simulink model "Cooling_System"  (R2019b)
settings: Solver=VariableStepAuto  StartTime=0.0  StopTime=3600  RelTol=1e-3
libraries: fl_lib x170, nesl_utility x49
(part 1 of 2)
settings Model: Creator=ZHOU Jinhan  LastModifiedBy=ZHOU Jinhan

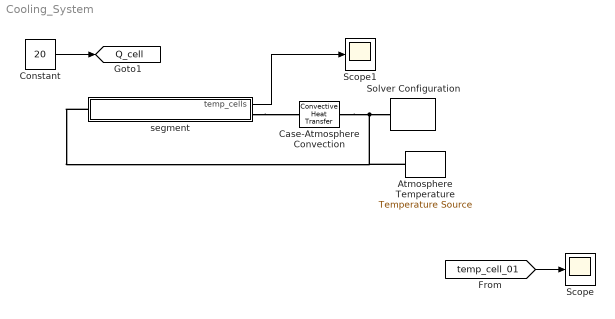
== system Cooling_System ==
  Atmosphere Temperature : fl_lib/Thermal/Thermal Sources/Temperature Source  temperature=25 degC
      settings: SourceProductName=Simscape
  Case-Atmosphere Convection : fl_lib/Thermal/Thermal Elements/Convective Heat Transfer  area=2160 cm^2  heat_tr_coeff=50 W/(m^2 * K)  T_specify=off  T_priority=None  T=0 K  T_nominal_specify=off  T_nominal_unit=K  T_nominal_value=1  Q_specify=off  Q_priority=None  Q=0 W  Q_nominal_specify=off  Q_nominal_unit=W  Q_nominal_value=1
  Constant : Constant  Value=20
  Scope : Scope
  Scope1 : Scope
  Solver Configuration : nesl_utility/Solver Configuration  PhysicalDomain=network_engine_domain  SubClassName=solver  LeftPortType=input  RightPortType=generic  Tones=[]  Harmonics=[]  SimulateNoise=off  Profile=off  UseLocalSampling=off  EnableSwitchedLinearOptims=on  FrequencyDomain=off  UseCCode=off  RelTol=0.001  AbsTol=1e-06  MinStep=1e-09  ToWorkspace=off  RevertToSquareIcSolve=off  NumHomotopyIterations=100  PhasorMode=off  PhasorModeNumHarmonics=1  DoDC=off  ResidualTolerance=1e-9  UseLocalSolver=off  LocalSolverChoice=NE_BACKWARD_EULER_ADVANCER  LocalSolverSampleTime=.001  DoFixedCost=off  MaxNonlinIter=3  MaxModeIter=2  LinearAlgebra=auto  EquationFormulation=NE_TIME_EF  DelaysMemoryBudget=1024  AutomaticFiltering=on  FilteringTimeConstant=0.001  PartitionStorageMethod=AS_NEEDED  PartitionMemoryBudget=1024  PartitionMethod=FAST
  segment : Subsystem
  tag scope: Q_cell=global
  wires:
  Constant/1 -> [Q_cell]
  [temp_cell_01] -> Scope/1
  segment/1(temp_cells) -> Scope1/1
  connections:
  segment/RConn1 -- Case-Atmosphere Convection/LConn1
  Case-Atmosphere Convection/RConn1 -- segment/LConn1 -- Atmosphere Temperature/LConn1 -- Solver Configuration/RConn1

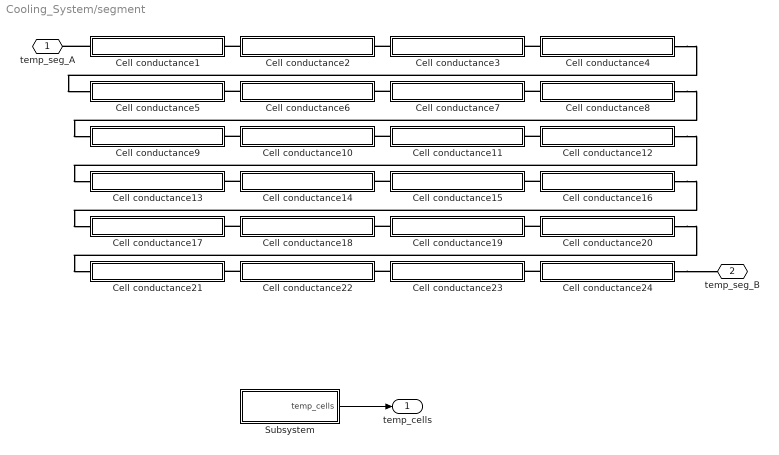
== system Cooling_System/segment ==
  Cell conductance1 : Subsystem
  Cell conductance10 : Subsystem
  Cell conductance11 : Subsystem
  Cell conductance12 : Subsystem
  Cell conductance13 : Subsystem
  Cell conductance14 : Subsystem
  Cell conductance15 : Subsystem
  Cell conductance16 : Subsystem
  Cell conductance17 : Subsystem
  Cell conductance18 : Subsystem
  "Cell conductance19 " : Subsystem
  Cell conductance2 : Subsystem
  Cell conductance20 : Subsystem
  Cell conductance21 : Subsystem
  Cell conductance22 : Subsystem
  Cell conductance23 : Subsystem
  Cell conductance24 : Subsystem
  Cell conductance3 : Subsystem
  Cell conductance4 : Subsystem
  Cell conductance5 : Subsystem
  Cell conductance6 : Subsystem
  Cell conductance7 : Subsystem
  Cell conductance8 : Subsystem
  Cell conductance9 : Subsystem
  Subsystem : Subsystem
  temp_seg_A : PMIOPort  Side=Left
  temp_seg_B : PMIOPort  Port=2  Side=Right
  temp_cells : Outport
  wires:
  Subsystem/1(temp_cells) -> temp_cells/1
  connections:
  Cell conductance2/LConn1 -- Cell conductance1/RConn1
  Cell conductance1/LConn1 -- temp_seg_A/RConn1
  Cell conductance24/RConn1 -- temp_seg_B/RConn1
  Cell conductance3/LConn1 -- Cell conductance2/RConn1
  Cell conductance4/LConn1 -- Cell conductance3/RConn1
  Cell conductance6/LConn1 -- Cell conductance5/RConn1
  Cell conductance7/LConn1 -- Cell conductance6/RConn1
  Cell conductance8/LConn1 -- Cell conductance7/RConn1
  Cell conductance10/LConn1 -- Cell conductance9/RConn1
  Cell conductance11/LConn1 -- Cell conductance10/RConn1
  Cell conductance12/LConn1 -- Cell conductance11/RConn1
  Cell conductance24/LConn1 -- Cell conductance23/RConn1
  Cell conductance23/LConn1 -- Cell conductance22/RConn1
  Cell conductance14/LConn1 -- Cell conductance13/RConn1
  Cell conductance18/LConn1 -- Cell conductance17/RConn1
  Cell conductance15/LConn1 -- Cell conductance14/RConn1
  Cell conductance16/LConn1 -- Cell conductance15/RConn1
  "Cell conductance19 "/LConn1 -- Cell conductance18/RConn1
  Cell conductance22/LConn1 -- Cell conductance21/RConn1
  Cell conductance20/LConn1 -- "Cell conductance19 "/RConn1
  Cell conductance4/RConn1 -- Cell conductance5/LConn1
  Cell conductance8/RConn1 -- Cell conductance9/LConn1
  Cell conductance12/RConn1 -- Cell conductance13/LConn1
  Cell conductance16/RConn1 -- Cell conductance17/LConn1
  Cell conductance20/RConn1 -- Cell conductance21/LConn1

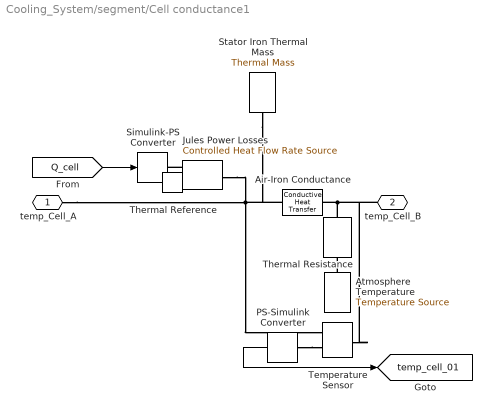
== system Cooling_System/segment/Cell conductance1 ==
  Air-Iron Conductance : fl_lib/Thermal/Thermal Elements/Conductive Heat Transfer  area=0.014 m^2  thickness=2 mm  th_cond=0.0257 W/(m*K)  T_specify=off  T_priority=None  T=0 K  T_nominal_specify=off  T_nominal_unit=K  T_nominal_value=1  Q_specify=off  Q_priority=None  Q=0 W  Q_nominal_specify=off  Q_nominal_unit=W  Q_nominal_value=1
      settings: SourceProductName=Simscape
  Atmosphere Temperature : fl_lib/Thermal/Thermal Sources/Temperature Source  temperature=300 K
      settings: SourceProductName=Simscape
  Jules Power Losses : fl_lib/Thermal/Thermal Sources/Controlled Heat Flow Rate Source
      settings: SourceProductName=Simscape
  PS-Simulink Converter : nesl_utility/PS-Simulink Converter  PhysicalDomain=network_engine_domain  SubClassName=ps_output  LeftPortType=input  RightPortType=output  PseudoPeriodic=off  Frequencies=[]  Unit=1  AffineConversion=off
  Simulink-PS Converter : nesl_utility/Simulink-PS Converter  PhysicalDomain=network_engine_domain  SubClassName=ps_input  LeftPortType=input  RightPortType=output  PseudoPeriodic=off  Frequencies=[]  NoiseDistribution=none  NoiseParameters=[]  Unit=W  AffineConversion=off  FilteringAndDerivatives=zero  SimscapeFilterOrder=1  InputFilterTimeConstant=.001  UdotUserProvided=[]
  Stator Iron Thermal Mass : fl_lib/Thermal/Thermal Elements/Thermal Mass  mass=0.3 kg  sp_heat=460 J/kg/K  T_specify=off  T_priority=High  T=300 K  T_nominal_specify=off  T_nominal_unit=K  T_nominal_value=1  Q_specify=off  Q_priority=None  Q=0 W  Q_nominal_specify=off  Q_nominal_unit=W  Q_nominal_value=1
  Temperature Sensor : fl_lib/Thermal/Thermal Sensors/Temperature Sensor
  Thermal Reference : fl_lib/Thermal/Thermal Elements/Thermal Reference
  Thermal Resistance : fl_lib/Thermal/Thermal Elements/Thermal Resistance  resistance=1/(1.006*1.202*0.028*50.4/60*1000) K/W  T_specify=off  T_priority=None  T=0 K  T_nominal_specify=off  T_nominal_unit=K  T_nominal_value=1  Q_specify=off  Q_priority=None  Q=0 W  Q_nominal_specify=off  Q_nominal_unit=W  Q_nominal_value=1
      settings: SourceProductName=Simscape  SourceProductBaseCode=SS
  temp_Cell_A : PMIOPort  Side=Left
  temp_Cell_B : PMIOPort  Port=2  Side=Right
  tag scope: temp_cell_01=global
  wires:
  [Q_cell] -> Simulink-PS Converter/1
  PS-Simulink Converter/1 -> [temp_cell_01]
  connections:
  temp_Cell_A/RConn1 -- Stator Iron Thermal Mass/LConn1 -- Air-Iron Conductance/LConn1 -- Jules Power Losses/LConn1 -- Temperature Sensor/RConn1
  Air-Iron Conductance/RConn1 -- Temperature Sensor/LConn1 -- temp_Cell_B/RConn1 -- Thermal Resistance/LConn1
  Atmosphere Temperature/LConn1 -- Thermal Resistance/RConn1
  Jules Power Losses/RConn1 -- Simulink-PS Converter/RConn1
  PS-Simulink Converter/LConn1 -- Temperature Sensor/RConn2
  Thermal Reference/LConn1 -- Jules Power Losses/RConn2

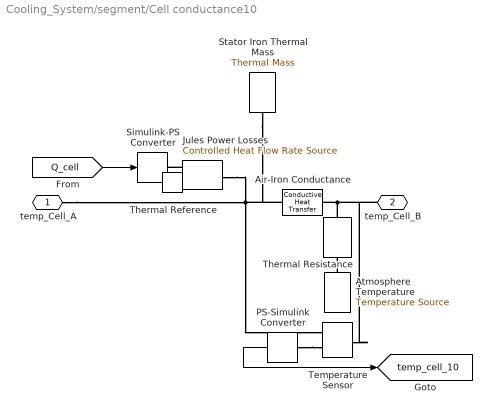
== system Cooling_System/segment/Cell conductance10 ==
  Air-Iron Conductance : fl_lib/Thermal/Thermal Elements/Conductive Heat Transfer  area=0.014 m^2  thickness=2 mm  th_cond=0.0257 W/(m*K)  T_specify=off  T_priority=None  T=0 K  T_nominal_specify=off  T_nominal_unit=K  T_nominal_value=1  Q_specify=off  Q_priority=None  Q=0 W  Q_nominal_specify=off  Q_nominal_unit=W  Q_nominal_value=1
      settings: SourceProductName=Simscape
  Atmosphere Temperature : fl_lib/Thermal/Thermal Sources/Temperature Source  temperature=300 K
      settings: SourceProductName=Simscape
  Jules Power Losses : fl_lib/Thermal/Thermal Sources/Controlled Heat Flow Rate Source
      settings: SourceProductName=Simscape
  PS-Simulink Converter : nesl_utility/PS-Simulink Converter  PhysicalDomain=network_engine_domain  SubClassName=ps_output  LeftPortType=input  RightPortType=output  PseudoPeriodic=off  Frequencies=[]  Unit=1  AffineConversion=off
  Simulink-PS Converter : nesl_utility/Simulink-PS Converter  PhysicalDomain=network_engine_domain  SubClassName=ps_input  LeftPortType=input  RightPortType=output  PseudoPeriodic=off  Frequencies=[]  NoiseDistribution=none  NoiseParameters=[]  Unit=W  AffineConversion=off  FilteringAndDerivatives=zero  SimscapeFilterOrder=1  InputFilterTimeConstant=.001  UdotUserProvided=[]
  Stator Iron Thermal Mass : fl_lib/Thermal/Thermal Elements/Thermal Mass  mass=0.3 kg  sp_heat=460 J/kg/K  T_specify=off  T_priority=High  T=300 K  T_nominal_specify=off  T_nominal_unit=K  T_nominal_value=1  Q_specify=off  Q_priority=None  Q=0 W  Q_nominal_specify=off  Q_nominal_unit=W  Q_nominal_value=1
  Temperature Sensor : fl_lib/Thermal/Thermal Sensors/Temperature Sensor
  Thermal Reference : fl_lib/Thermal/Thermal Elements/Thermal Reference
  Thermal Resistance : fl_lib/Thermal/Thermal Elements/Thermal Resistance  resistance=1/(1.006*1.202*0.028*50.4/60*1000) K/W  T_specify=off  T_priority=None  T=0 K  T_nominal_specify=off  T_nominal_unit=K  T_nominal_value=1  Q_specify=off  Q_priority=None  Q=0 W  Q_nominal_specify=off  Q_nominal_unit=W  Q_nominal_value=1
      settings: SourceProductName=Simscape  SourceProductBaseCode=SS
  temp_Cell_A : PMIOPort  Side=Left
  temp_Cell_B : PMIOPort  Port=2  Side=Right
  tag scope: temp_cell_10=global
  wires:
  [Q_cell] -> Simulink-PS Converter/1
  PS-Simulink Converter/1 -> [temp_cell_10]
  connections:
  Jules Power Losses/LConn1 -- temp_Cell_A/RConn1 -- Temperature Sensor/RConn1 -- Stator Iron Thermal Mass/LConn1 -- Air-Iron Conductance/LConn1
  Air-Iron Conductance/RConn1 -- Thermal Resistance/LConn1 -- temp_Cell_B/RConn1 -- Temperature Sensor/LConn1
  Atmosphere Temperature/LConn1 -- Thermal Resistance/RConn1
  Jules Power Losses/RConn1 -- Simulink-PS Converter/RConn1
  PS-Simulink Converter/LConn1 -- Temperature Sensor/RConn2
  Thermal Reference/LConn1 -- Jules Power Losses/RConn2

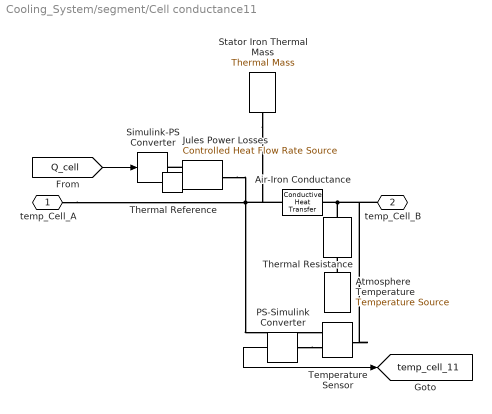
== system Cooling_System/segment/Cell conductance11 ==
  Air-Iron Conductance : fl_lib/Thermal/Thermal Elements/Conductive Heat Transfer  area=0.014 m^2  thickness=2 mm  th_cond=0.0257 W/(m*K)  T_specify=off  T_priority=None  T=0 K  T_nominal_specify=off  T_nominal_unit=K  T_nominal_value=1  Q_specify=off  Q_priority=None  Q=0 W  Q_nominal_specify=off  Q_nominal_unit=W  Q_nominal_value=1
      settings: SourceProductName=Simscape
  Atmosphere Temperature : fl_lib/Thermal/Thermal Sources/Temperature Source  temperature=300 K
      settings: SourceProductName=Simscape
  Jules Power Losses : fl_lib/Thermal/Thermal Sources/Controlled Heat Flow Rate Source
      settings: SourceProductName=Simscape
  PS-Simulink Converter : nesl_utility/PS-Simulink Converter  PhysicalDomain=network_engine_domain  SubClassName=ps_output  LeftPortType=input  RightPortType=output  PseudoPeriodic=off  Frequencies=[]  Unit=1  AffineConversion=off
  Simulink-PS Converter : nesl_utility/Simulink-PS Converter  PhysicalDomain=network_engine_domain  SubClassName=ps_input  LeftPortType=input  RightPortType=output  PseudoPeriodic=off  Frequencies=[]  NoiseDistribution=none  NoiseParameters=[]  Unit=W  AffineConversion=off  FilteringAndDerivatives=zero  SimscapeFilterOrder=1  InputFilterTimeConstant=.001  UdotUserProvided=[]
  Stator Iron Thermal Mass : fl_lib/Thermal/Thermal Elements/Thermal Mass  mass=0.3 kg  sp_heat=460 J/kg/K  T_specify=off  T_priority=High  T=300 K  T_nominal_specify=off  T_nominal_unit=K  T_nominal_value=1  Q_specify=off  Q_priority=None  Q=0 W  Q_nominal_specify=off  Q_nominal_unit=W  Q_nominal_value=1
  Temperature Sensor : fl_lib/Thermal/Thermal Sensors/Temperature Sensor
  Thermal Reference : fl_lib/Thermal/Thermal Elements/Thermal Reference
  Thermal Resistance : fl_lib/Thermal/Thermal Elements/Thermal Resistance  resistance=1/(1.006*1.202*0.028*50.4/60*1000) K/W  T_specify=off  T_priority=None  T=0 K  T_nominal_specify=off  T_nominal_unit=K  T_nominal_value=1  Q_specify=off  Q_priority=None  Q=0 W  Q_nominal_specify=off  Q_nominal_unit=W  Q_nominal_value=1
      settings: SourceProductName=Simscape  SourceProductBaseCode=SS
  temp_Cell_A : PMIOPort  Side=Left
  temp_Cell_B : PMIOPort  Port=2  Side=Right
  tag scope: temp_cell_11=global
  wires:
  [Q_cell] -> Simulink-PS Converter/1
  PS-Simulink Converter/1 -> [temp_cell_11]
  connections:
  Jules Power Losses/LConn1 -- temp_Cell_A/RConn1 -- Temperature Sensor/RConn1 -- Stator Iron Thermal Mass/LConn1 -- Air-Iron Conductance/LConn1
  Air-Iron Conductance/RConn1 -- Thermal Resistance/LConn1 -- temp_Cell_B/RConn1 -- Temperature Sensor/LConn1
  Atmosphere Temperature/LConn1 -- Thermal Resistance/RConn1
  Jules Power Losses/RConn1 -- Simulink-PS Converter/RConn1
  PS-Simulink Converter/LConn1 -- Temperature Sensor/RConn2
  Thermal Reference/LConn1 -- Jules Power Losses/RConn2

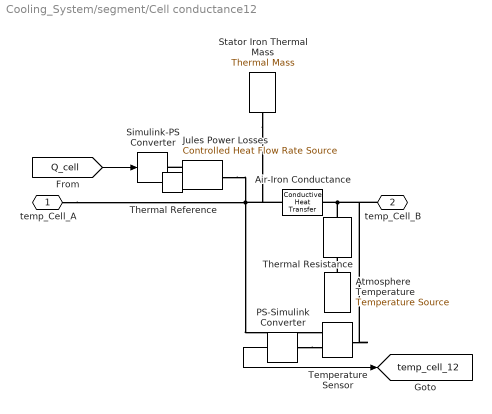
== system Cooling_System/segment/Cell conductance12 ==
  Air-Iron Conductance : fl_lib/Thermal/Thermal Elements/Conductive Heat Transfer  area=0.014 m^2  thickness=2 mm  th_cond=0.0257 W/(m*K)  T_specify=off  T_priority=None  T=0 K  T_nominal_specify=off  T_nominal_unit=K  T_nominal_value=1  Q_specify=off  Q_priority=None  Q=0 W  Q_nominal_specify=off  Q_nominal_unit=W  Q_nominal_value=1
      settings: SourceProductName=Simscape
  Atmosphere Temperature : fl_lib/Thermal/Thermal Sources/Temperature Source  temperature=300 K
      settings: SourceProductName=Simscape
  Jules Power Losses : fl_lib/Thermal/Thermal Sources/Controlled Heat Flow Rate Source
      settings: SourceProductName=Simscape
  PS-Simulink Converter : nesl_utility/PS-Simulink Converter  PhysicalDomain=network_engine_domain  SubClassName=ps_output  LeftPortType=input  RightPortType=output  PseudoPeriodic=off  Frequencies=[]  Unit=1  AffineConversion=off
  Simulink-PS Converter : nesl_utility/Simulink-PS Converter  PhysicalDomain=network_engine_domain  SubClassName=ps_input  LeftPortType=input  RightPortType=output  PseudoPeriodic=off  Frequencies=[]  NoiseDistribution=none  NoiseParameters=[]  Unit=W  AffineConversion=off  FilteringAndDerivatives=zero  SimscapeFilterOrder=1  InputFilterTimeConstant=.001  UdotUserProvided=[]
  Stator Iron Thermal Mass : fl_lib/Thermal/Thermal Elements/Thermal Mass  mass=0.3 kg  sp_heat=460 J/kg/K  T_specify=off  T_priority=High  T=300 K  T_nominal_specify=off  T_nominal_unit=K  T_nominal_value=1  Q_specify=off  Q_priority=None  Q=0 W  Q_nominal_specify=off  Q_nominal_unit=W  Q_nominal_value=1
  Temperature Sensor : fl_lib/Thermal/Thermal Sensors/Temperature Sensor
  Thermal Reference : fl_lib/Thermal/Thermal Elements/Thermal Reference
  Thermal Resistance : fl_lib/Thermal/Thermal Elements/Thermal Resistance  resistance=1/(1.006*1.202*0.028*50.4/60*1000) K/W  T_specify=off  T_priority=None  T=0 K  T_nominal_specify=off  T_nominal_unit=K  T_nominal_value=1  Q_specify=off  Q_priority=None  Q=0 W  Q_nominal_specify=off  Q_nominal_unit=W  Q_nominal_value=1
      settings: SourceProductName=Simscape  SourceProductBaseCode=SS
  temp_Cell_A : PMIOPort  Side=Left
  temp_Cell_B : PMIOPort  Port=2  Side=Right
  tag scope: temp_cell_12=global
  wires:
  [Q_cell] -> Simulink-PS Converter/1
  PS-Simulink Converter/1 -> [temp_cell_12]
  connections:
  Jules Power Losses/LConn1 -- temp_Cell_A/RConn1 -- Temperature Sensor/RConn1 -- Stator Iron Thermal Mass/LConn1 -- Air-Iron Conductance/LConn1
  Air-Iron Conductance/RConn1 -- Thermal Resistance/LConn1 -- temp_Cell_B/RConn1 -- Temperature Sensor/LConn1
  Atmosphere Temperature/LConn1 -- Thermal Resistance/RConn1
  Jules Power Losses/RConn1 -- Simulink-PS Converter/RConn1
  PS-Simulink Converter/LConn1 -- Temperature Sensor/RConn2
  Thermal Reference/LConn1 -- Jules Power Losses/RConn2

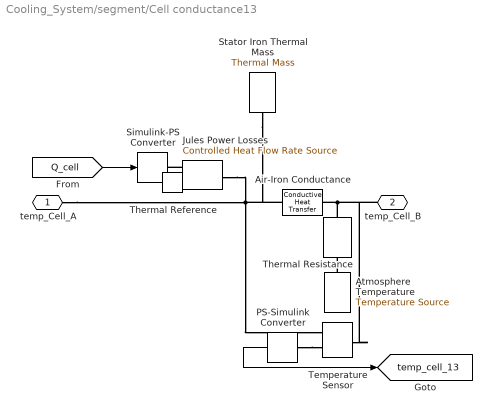
== system Cooling_System/segment/Cell conductance13 ==
  Air-Iron Conductance : fl_lib/Thermal/Thermal Elements/Conductive Heat Transfer  area=0.014 m^2  thickness=2 mm  th_cond=0.0257 W/(m*K)  T_specify=off  T_priority=None  T=0 K  T_nominal_specify=off  T_nominal_unit=K  T_nominal_value=1  Q_specify=off  Q_priority=None  Q=0 W  Q_nominal_specify=off  Q_nominal_unit=W  Q_nominal_value=1
      settings: SourceProductName=Simscape
  Atmosphere Temperature : fl_lib/Thermal/Thermal Sources/Temperature Source  temperature=300 K
      settings: SourceProductName=Simscape
  Jules Power Losses : fl_lib/Thermal/Thermal Sources/Controlled Heat Flow Rate Source
      settings: SourceProductName=Simscape
  PS-Simulink Converter : nesl_utility/PS-Simulink Converter  PhysicalDomain=network_engine_domain  SubClassName=ps_output  LeftPortType=input  RightPortType=output  PseudoPeriodic=off  Frequencies=[]  Unit=1  AffineConversion=off
  Simulink-PS Converter : nesl_utility/Simulink-PS Converter  PhysicalDomain=network_engine_domain  SubClassName=ps_input  LeftPortType=input  RightPortType=output  PseudoPeriodic=off  Frequencies=[]  NoiseDistribution=none  NoiseParameters=[]  Unit=W  AffineConversion=off  FilteringAndDerivatives=zero  SimscapeFilterOrder=1  InputFilterTimeConstant=.001  UdotUserProvided=[]
  Stator Iron Thermal Mass : fl_lib/Thermal/Thermal Elements/Thermal Mass  mass=0.3 kg  sp_heat=460 J/kg/K  T_specify=off  T_priority=High  T=300 K  T_nominal_specify=off  T_nominal_unit=K  T_nominal_value=1  Q_specify=off  Q_priority=None  Q=0 W  Q_nominal_specify=off  Q_nominal_unit=W  Q_nominal_value=1
  Temperature Sensor : fl_lib/Thermal/Thermal Sensors/Temperature Sensor
  Thermal Reference : fl_lib/Thermal/Thermal Elements/Thermal Reference
  Thermal Resistance : fl_lib/Thermal/Thermal Elements/Thermal Resistance  resistance=1/(1.006*1.202*0.028*50.4/60*1000) K/W  T_specify=off  T_priority=None  T=0 K  T_nominal_specify=off  T_nominal_unit=K  T_nominal_value=1  Q_specify=off  Q_priority=None  Q=0 W  Q_nominal_specify=off  Q_nominal_unit=W  Q_nominal_value=1
      settings: SourceProductName=Simscape  SourceProductBaseCode=SS
  temp_Cell_A : PMIOPort  Side=Left
  temp_Cell_B : PMIOPort  Port=2  Side=Right
  tag scope: temp_cell_13=global
  wires:
  [Q_cell] -> Simulink-PS Converter/1
  PS-Simulink Converter/1 -> [temp_cell_13]
  connections:
  Jules Power Losses/LConn1 -- temp_Cell_A/RConn1 -- Temperature Sensor/RConn1 -- Stator Iron Thermal Mass/LConn1 -- Air-Iron Conductance/LConn1
  Air-Iron Conductance/RConn1 -- Thermal Resistance/LConn1 -- temp_Cell_B/RConn1 -- Temperature Sensor/LConn1
  Atmosphere Temperature/LConn1 -- Thermal Resistance/RConn1
  Jules Power Losses/RConn1 -- Simulink-PS Converter/RConn1
  PS-Simulink Converter/LConn1 -- Temperature Sensor/RConn2
  Thermal Reference/LConn1 -- Jules Power Losses/RConn2

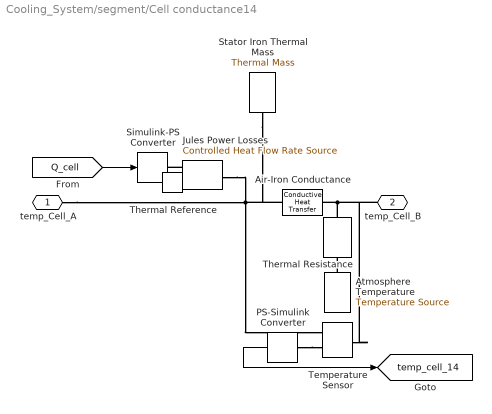
== system Cooling_System/segment/Cell conductance14 ==
  Air-Iron Conductance : fl_lib/Thermal/Thermal Elements/Conductive Heat Transfer  area=0.014 m^2  thickness=2 mm  th_cond=0.0257 W/(m*K)  T_specify=off  T_priority=None  T=0 K  T_nominal_specify=off  T_nominal_unit=K  T_nominal_value=1  Q_specify=off  Q_priority=None  Q=0 W  Q_nominal_specify=off  Q_nominal_unit=W  Q_nominal_value=1
      settings: SourceProductName=Simscape
  Atmosphere Temperature : fl_lib/Thermal/Thermal Sources/Temperature Source  temperature=300 K
      settings: SourceProductName=Simscape
  Jules Power Losses : fl_lib/Thermal/Thermal Sources/Controlled Heat Flow Rate Source
      settings: SourceProductName=Simscape
  PS-Simulink Converter : nesl_utility/PS-Simulink Converter  PhysicalDomain=network_engine_domain  SubClassName=ps_output  LeftPortType=input  RightPortType=output  PseudoPeriodic=off  Frequencies=[]  Unit=1  AffineConversion=off
  Simulink-PS Converter : nesl_utility/Simulink-PS Converter  PhysicalDomain=network_engine_domain  SubClassName=ps_input  LeftPortType=input  RightPortType=output  PseudoPeriodic=off  Frequencies=[]  NoiseDistribution=none  NoiseParameters=[]  Unit=W  AffineConversion=off  FilteringAndDerivatives=zero  SimscapeFilterOrder=1  InputFilterTimeConstant=.001  UdotUserProvided=[]
  Stator Iron Thermal Mass : fl_lib/Thermal/Thermal Elements/Thermal Mass  mass=0.3 kg  sp_heat=460 J/kg/K  T_specify=off  T_priority=High  T=300 K  T_nominal_specify=off  T_nominal_unit=K  T_nominal_value=1  Q_specify=off  Q_priority=None  Q=0 W  Q_nominal_specify=off  Q_nominal_unit=W  Q_nominal_value=1
  Temperature Sensor : fl_lib/Thermal/Thermal Sensors/Temperature Sensor
  Thermal Reference : fl_lib/Thermal/Thermal Elements/Thermal Reference
  Thermal Resistance : fl_lib/Thermal/Thermal Elements/Thermal Resistance  resistance=1/(1.006*1.202*0.028*50.4/60*1000) K/W  T_specify=off  T_priority=None  T=0 K  T_nominal_specify=off  T_nominal_unit=K  T_nominal_value=1  Q_specify=off  Q_priority=None  Q=0 W  Q_nominal_specify=off  Q_nominal_unit=W  Q_nominal_value=1
      settings: SourceProductName=Simscape  SourceProductBaseCode=SS
  temp_Cell_A : PMIOPort  Side=Left
  temp_Cell_B : PMIOPort  Port=2  Side=Right
  tag scope: temp_cell_14=global
  wires:
  [Q_cell] -> Simulink-PS Converter/1
  PS-Simulink Converter/1 -> [temp_cell_14]
  connections:
  Jules Power Losses/LConn1 -- temp_Cell_A/RConn1 -- Temperature Sensor/RConn1 -- Stator Iron Thermal Mass/LConn1 -- Air-Iron Conductance/LConn1
  Air-Iron Conductance/RConn1 -- Thermal Resistance/LConn1 -- temp_Cell_B/RConn1 -- Temperature Sensor/LConn1
  Atmosphere Temperature/LConn1 -- Thermal Resistance/RConn1
  Jules Power Losses/RConn1 -- Simulink-PS Converter/RConn1
  PS-Simulink Converter/LConn1 -- Temperature Sensor/RConn2
  Thermal Reference/LConn1 -- Jules Power Losses/RConn2

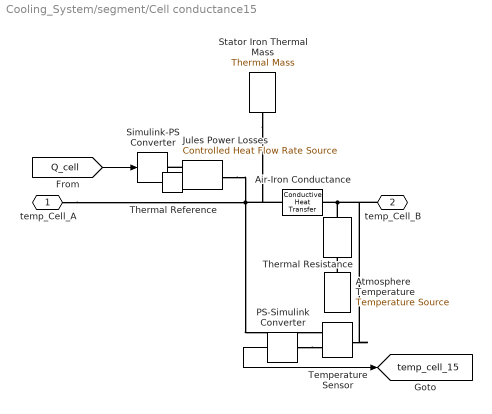
== system Cooling_System/segment/Cell conductance15 ==
  Air-Iron Conductance : fl_lib/Thermal/Thermal Elements/Conductive Heat Transfer  area=0.014 m^2  thickness=2 mm  th_cond=0.0257 W/(m*K)  T_specify=off  T_priority=None  T=0 K  T_nominal_specify=off  T_nominal_unit=K  T_nominal_value=1  Q_specify=off  Q_priority=None  Q=0 W  Q_nominal_specify=off  Q_nominal_unit=W  Q_nominal_value=1
      settings: SourceProductName=Simscape
  Atmosphere Temperature : fl_lib/Thermal/Thermal Sources/Temperature Source  temperature=300 K
      settings: SourceProductName=Simscape
  Jules Power Losses : fl_lib/Thermal/Thermal Sources/Controlled Heat Flow Rate Source
      settings: SourceProductName=Simscape
  PS-Simulink Converter : nesl_utility/PS-Simulink Converter  PhysicalDomain=network_engine_domain  SubClassName=ps_output  LeftPortType=input  RightPortType=output  PseudoPeriodic=off  Frequencies=[]  Unit=1  AffineConversion=off
  Simulink-PS Converter : nesl_utility/Simulink-PS Converter  PhysicalDomain=network_engine_domain  SubClassName=ps_input  LeftPortType=input  RightPortType=output  PseudoPeriodic=off  Frequencies=[]  NoiseDistribution=none  NoiseParameters=[]  Unit=W  AffineConversion=off  FilteringAndDerivatives=zero  SimscapeFilterOrder=1  InputFilterTimeConstant=.001  UdotUserProvided=[]
  Stator Iron Thermal Mass : fl_lib/Thermal/Thermal Elements/Thermal Mass  mass=0.3 kg  sp_heat=460 J/kg/K  T_specify=off  T_priority=High  T=300 K  T_nominal_specify=off  T_nominal_unit=K  T_nominal_value=1  Q_specify=off  Q_priority=None  Q=0 W  Q_nominal_specify=off  Q_nominal_unit=W  Q_nominal_value=1
  Temperature Sensor : fl_lib/Thermal/Thermal Sensors/Temperature Sensor
  Thermal Reference : fl_lib/Thermal/Thermal Elements/Thermal Reference
  Thermal Resistance : fl_lib/Thermal/Thermal Elements/Thermal Resistance  resistance=1/(1.006*1.202*0.028*50.4/60*1000) K/W  T_specify=off  T_priority=None  T=0 K  T_nominal_specify=off  T_nominal_unit=K  T_nominal_value=1  Q_specify=off  Q_priority=None  Q=0 W  Q_nominal_specify=off  Q_nominal_unit=W  Q_nominal_value=1
      settings: SourceProductName=Simscape  SourceProductBaseCode=SS
  temp_Cell_A : PMIOPort  Side=Left
  temp_Cell_B : PMIOPort  Port=2  Side=Right
  tag scope: temp_cell_15=global
  wires:
  [Q_cell] -> Simulink-PS Converter/1
  PS-Simulink Converter/1 -> [temp_cell_15]
  connections:
  Jules Power Losses/LConn1 -- temp_Cell_A/RConn1 -- Temperature Sensor/RConn1 -- Stator Iron Thermal Mass/LConn1 -- Air-Iron Conductance/LConn1
  Air-Iron Conductance/RConn1 -- Thermal Resistance/LConn1 -- temp_Cell_B/RConn1 -- Temperature Sensor/LConn1
  Atmosphere Temperature/LConn1 -- Thermal Resistance/RConn1
  Jules Power Losses/RConn1 -- Simulink-PS Converter/RConn1
  PS-Simulink Converter/LConn1 -- Temperature Sensor/RConn2
  Thermal Reference/LConn1 -- Jules Power Losses/RConn2

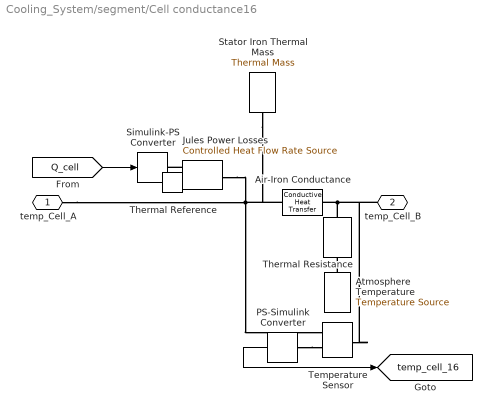
== system Cooling_System/segment/Cell conductance16 ==
  Air-Iron Conductance : fl_lib/Thermal/Thermal Elements/Conductive Heat Transfer  area=0.014 m^2  thickness=2 mm  th_cond=0.0257 W/(m*K)  T_specify=off  T_priority=None  T=0 K  T_nominal_specify=off  T_nominal_unit=K  T_nominal_value=1  Q_specify=off  Q_priority=None  Q=0 W  Q_nominal_specify=off  Q_nominal_unit=W  Q_nominal_value=1
      settings: SourceProductName=Simscape
  Atmosphere Temperature : fl_lib/Thermal/Thermal Sources/Temperature Source  temperature=300 K
      settings: SourceProductName=Simscape
  Jules Power Losses : fl_lib/Thermal/Thermal Sources/Controlled Heat Flow Rate Source
      settings: SourceProductName=Simscape
  PS-Simulink Converter : nesl_utility/PS-Simulink Converter  PhysicalDomain=network_engine_domain  SubClassName=ps_output  LeftPortType=input  RightPortType=output  PseudoPeriodic=off  Frequencies=[]  Unit=1  AffineConversion=off
  Simulink-PS Converter : nesl_utility/Simulink-PS Converter  PhysicalDomain=network_engine_domain  SubClassName=ps_input  LeftPortType=input  RightPortType=output  PseudoPeriodic=off  Frequencies=[]  NoiseDistribution=none  NoiseParameters=[]  Unit=W  AffineConversion=off  FilteringAndDerivatives=zero  SimscapeFilterOrder=1  InputFilterTimeConstant=.001  UdotUserProvided=[]
  Stator Iron Thermal Mass : fl_lib/Thermal/Thermal Elements/Thermal Mass  mass=0.3 kg  sp_heat=460 J/kg/K  T_specify=off  T_priority=High  T=300 K  T_nominal_specify=off  T_nominal_unit=K  T_nominal_value=1  Q_specify=off  Q_priority=None  Q=0 W  Q_nominal_specify=off  Q_nominal_unit=W  Q_nominal_value=1
  Temperature Sensor : fl_lib/Thermal/Thermal Sensors/Temperature Sensor
  Thermal Reference : fl_lib/Thermal/Thermal Elements/Thermal Reference
  Thermal Resistance : fl_lib/Thermal/Thermal Elements/Thermal Resistance  resistance=1/(1.006*1.202*0.028*50.4/60*1000) K/W  T_specify=off  T_priority=None  T=0 K  T_nominal_specify=off  T_nominal_unit=K  T_nominal_value=1  Q_specify=off  Q_priority=None  Q=0 W  Q_nominal_specify=off  Q_nominal_unit=W  Q_nominal_value=1
      settings: SourceProductName=Simscape  SourceProductBaseCode=SS
  temp_Cell_A : PMIOPort  Side=Left
  temp_Cell_B : PMIOPort  Port=2  Side=Right
  tag scope: temp_cell_16=global
  wires:
  [Q_cell] -> Simulink-PS Converter/1
  PS-Simulink Converter/1 -> [temp_cell_16]
  connections:
  Jules Power Losses/LConn1 -- temp_Cell_A/RConn1 -- Temperature Sensor/RConn1 -- Stator Iron Thermal Mass/LConn1 -- Air-Iron Conductance/LConn1
  Air-Iron Conductance/RConn1 -- Thermal Resistance/LConn1 -- temp_Cell_B/RConn1 -- Temperature Sensor/LConn1
  Atmosphere Temperature/LConn1 -- Thermal Resistance/RConn1
  Jules Power Losses/RConn1 -- Simulink-PS Converter/RConn1
  PS-Simulink Converter/LConn1 -- Temperature Sensor/RConn2
  Thermal Reference/LConn1 -- Jules Power Losses/RConn2

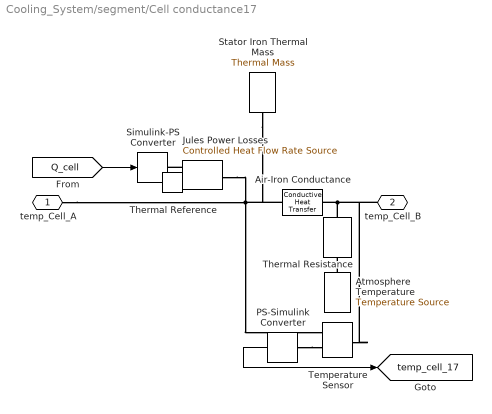
== system Cooling_System/segment/Cell conductance17 ==
  Air-Iron Conductance : fl_lib/Thermal/Thermal Elements/Conductive Heat Transfer  area=0.014 m^2  thickness=2 mm  th_cond=0.0257 W/(m*K)  T_specify=off  T_priority=None  T=0 K  T_nominal_specify=off  T_nominal_unit=K  T_nominal_value=1  Q_specify=off  Q_priority=None  Q=0 W  Q_nominal_specify=off  Q_nominal_unit=W  Q_nominal_value=1
      settings: SourceProductName=Simscape
  Atmosphere Temperature : fl_lib/Thermal/Thermal Sources/Temperature Source  temperature=300 K
      settings: SourceProductName=Simscape
  Jules Power Losses : fl_lib/Thermal/Thermal Sources/Controlled Heat Flow Rate Source
      settings: SourceProductName=Simscape
  PS-Simulink Converter : nesl_utility/PS-Simulink Converter  PhysicalDomain=network_engine_domain  SubClassName=ps_output  LeftPortType=input  RightPortType=output  PseudoPeriodic=off  Frequencies=[]  Unit=1  AffineConversion=off
  Simulink-PS Converter : nesl_utility/Simulink-PS Converter  PhysicalDomain=network_engine_domain  SubClassName=ps_input  LeftPortType=input  RightPortType=output  PseudoPeriodic=off  Frequencies=[]  NoiseDistribution=none  NoiseParameters=[]  Unit=W  AffineConversion=off  FilteringAndDerivatives=zero  SimscapeFilterOrder=1  InputFilterTimeConstant=.001  UdotUserProvided=[]
  Stator Iron Thermal Mass : fl_lib/Thermal/Thermal Elements/Thermal Mass  mass=0.3 kg  sp_heat=460 J/kg/K  T_specify=off  T_priority=High  T=300 K  T_nominal_specify=off  T_nominal_unit=K  T_nominal_value=1  Q_specify=off  Q_priority=None  Q=0 W  Q_nominal_specify=off  Q_nominal_unit=W  Q_nominal_value=1
  Temperature Sensor : fl_lib/Thermal/Thermal Sensors/Temperature Sensor
  Thermal Reference : fl_lib/Thermal/Thermal Elements/Thermal Reference
  Thermal Resistance : fl_lib/Thermal/Thermal Elements/Thermal Resistance  resistance=1/(1.006*1.202*0.028*50.4/60*1000) K/W  T_specify=off  T_priority=None  T=0 K  T_nominal_specify=off  T_nominal_unit=K  T_nominal_value=1  Q_specify=off  Q_priority=None  Q=0 W  Q_nominal_specify=off  Q_nominal_unit=W  Q_nominal_value=1
      settings: SourceProductName=Simscape  SourceProductBaseCode=SS
  temp_Cell_A : PMIOPort  Side=Left
  temp_Cell_B : PMIOPort  Port=2  Side=Right
  tag scope: temp_cell_17=global
  wires:
  [Q_cell] -> Simulink-PS Converter/1
  PS-Simulink Converter/1 -> [temp_cell_17]
  connections:
  Jules Power Losses/LConn1 -- temp_Cell_A/RConn1 -- Temperature Sensor/RConn1 -- Stator Iron Thermal Mass/LConn1 -- Air-Iron Conductance/LConn1
  Air-Iron Conductance/RConn1 -- Thermal Resistance/LConn1 -- temp_Cell_B/RConn1 -- Temperature Sensor/LConn1
  Atmosphere Temperature/LConn1 -- Thermal Resistance/RConn1
  Jules Power Losses/RConn1 -- Simulink-PS Converter/RConn1
  PS-Simulink Converter/LConn1 -- Temperature Sensor/RConn2
  Thermal Reference/LConn1 -- Jules Power Losses/RConn2

== system Cooling_System/segment/Cell conductance18 ==
  Air-Iron Conductance : fl_lib/Thermal/Thermal Elements/Conductive Heat Transfer  area=0.014 m^2  thickness=2 mm  th_cond=0.0257 W/(m*K)  T_specify=off  T_priority=None  T=0 K  T_nominal_specify=off  T_nominal_unit=K  T_nominal_value=1  Q_specify=off  Q_priority=None  Q=0 W  Q_nominal_specify=off  Q_nominal_unit=W  Q_nominal_value=1
      settings: SourceProductName=Simscape
  Atmosphere Temperature : fl_lib/Thermal/Thermal Sources/Temperature Source  temperature=300 K
      settings: SourceProductName=Simscape
  Jules Power Losses : fl_lib/Thermal/Thermal Sources/Controlled Heat Flow Rate Source
      settings: SourceProductName=Simscape
  PS-Simulink Converter : nesl_utility/PS-Simulink Converter  PhysicalDomain=network_engine_domain  SubClassName=ps_output  LeftPortType=input  RightPortType=output  PseudoPeriodic=off  Frequencies=[]  Unit=1  AffineConversion=off
  Simulink-PS Converter : nesl_utility/Simulink-PS Converter  PhysicalDomain=network_engine_domain  SubClassName=ps_input  LeftPortType=input  RightPortType=output  PseudoPeriodic=off  Frequencies=[]  NoiseDistribution=none  NoiseParameters=[]  Unit=W  AffineConversion=off  FilteringAndDerivatives=zero  SimscapeFilterOrder=1  InputFilterTimeConstant=.001  UdotUserProvided=[]
  Stator Iron Thermal Mass : fl_lib/Thermal/Thermal Elements/Thermal Mass  mass=0.3 kg  sp_heat=460 J/kg/K  T_specify=off  T_priority=High  T=300 K  T_nominal_specify=off  T_nominal_unit=K  T_nominal_value=1  Q_specify=off  Q_priority=None  Q=0 W  Q_nominal_specify=off  Q_nominal_unit=W  Q_nominal_value=1
  Temperature Sensor : fl_lib/Thermal/Thermal Sensors/Temperature Sensor
  Thermal Reference : fl_lib/Thermal/Thermal Elements/Thermal Reference
  Thermal Resistance : fl_lib/Thermal/Thermal Elements/Thermal Resistance  resistance=1/(1.006*1.202*0.028*50.4/60*1000) K/W  T_specify=off  T_priority=None  T=0 K  T_nominal_specify=off  T_nominal_unit=K  T_nominal_value=1  Q_specify=off  Q_priority=None  Q=0 W  Q_nominal_specify=off  Q_nominal_unit=W  Q_nominal_value=1
      settings: SourceProductName=Simscape  SourceProductBaseCode=SS
  temp_Cell_A : PMIOPort  Side=Left
  temp_Cell_B : PMIOPort  Port=2  Side=Right
  tag scope: temp_cell_18=global
  wires:
  [Q_cell] -> Simulink-PS Converter/1
  PS-Simulink Converter/1 -> [temp_cell_18]
  connections:
  Jules Power Losses/LConn1 -- temp_Cell_A/RConn1 -- Temperature Sensor/RConn1 -- Stator Iron Thermal Mass/LConn1 -- Air-Iron Conductance/LConn1
  Air-Iron Conductance/RConn1 -- Thermal Resistance/LConn1 -- temp_Cell_B/RConn1 -- Temperature Sensor/LConn1
  Atmosphere Temperature/LConn1 -- Thermal Resistance/RConn1
  Jules Power Losses/RConn1 -- Simulink-PS Converter/RConn1
  PS-Simulink Converter/LConn1 -- Temperature Sensor/RConn2
  Thermal Reference/LConn1 -- Jules Power Losses/RConn2

== system Cooling_System/segment/Cell conductance19  ==
  Air-Iron Conductance : fl_lib/Thermal/Thermal Elements/Conductive Heat Transfer  area=0.014 m^2  thickness=2 mm  th_cond=0.0257 W/(m*K)  T_specify=off  T_priority=None  T=0 K  T_nominal_specify=off  T_nominal_unit=K  T_nominal_value=1  Q_specify=off  Q_priority=None  Q=0 W  Q_nominal_specify=off  Q_nominal_unit=W  Q_nominal_value=1
      settings: SourceProductName=Simscape
  Atmosphere Temperature : fl_lib/Thermal/Thermal Sources/Temperature Source  temperature=300 K
      settings: SourceProductName=Simscape
  Jules Power Losses : fl_lib/Thermal/Thermal Sources/Controlled Heat Flow Rate Source
      settings: SourceProductName=Simscape
  PS-Simulink Converter : nesl_utility/PS-Simulink Converter  PhysicalDomain=network_engine_domain  SubClassName=ps_output  LeftPortType=input  RightPortType=output  PseudoPeriodic=off  Frequencies=[]  Unit=1  AffineConversion=off
  Simulink-PS Converter : nesl_utility/Simulink-PS Converter  PhysicalDomain=network_engine_domain  SubClassName=ps_input  LeftPortType=input  RightPortType=output  PseudoPeriodic=off  Frequencies=[]  NoiseDistribution=none  NoiseParameters=[]  Unit=W  AffineConversion=off  FilteringAndDerivatives=zero  SimscapeFilterOrder=1  InputFilterTimeConstant=.001  UdotUserProvided=[]
  Stator Iron Thermal Mass : fl_lib/Thermal/Thermal Elements/Thermal Mass  mass=0.3 kg  sp_heat=460 J/kg/K  T_specify=off  T_priority=High  T=300 K  T_nominal_specify=off  T_nominal_unit=K  T_nominal_value=1  Q_specify=off  Q_priority=None  Q=0 W  Q_nominal_specify=off  Q_nominal_unit=W  Q_nominal_value=1
  Temperature Sensor : fl_lib/Thermal/Thermal Sensors/Temperature Sensor
  Thermal Reference : fl_lib/Thermal/Thermal Elements/Thermal Reference
  Thermal Resistance : fl_lib/Thermal/Thermal Elements/Thermal Resistance  resistance=1/(1.006*1.202*0.028*50.4/60*1000) K/W  T_specify=off  T_priority=None  T=0 K  T_nominal_specify=off  T_nominal_unit=K  T_nominal_value=1  Q_specify=off  Q_priority=None  Q=0 W  Q_nominal_specify=off  Q_nominal_unit=W  Q_nominal_value=1
      settings: SourceProductName=Simscape  SourceProductBaseCode=SS
  temp_Cell_A : PMIOPort  Side=Left
  temp_Cell_B : PMIOPort  Port=2  Side=Right
  tag scope: temp_cell_19=global
  wires:
  [Q_cell] -> Simulink-PS Converter/1
  PS-Simulink Converter/1 -> [temp_cell_19]
  connections:
  Jules Power Losses/LConn1 -- temp_Cell_A/RConn1 -- Temperature Sensor/RConn1 -- Stator Iron Thermal Mass/LConn1 -- Air-Iron Conductance/LConn1
  Air-Iron Conductance/RConn1 -- Thermal Resistance/LConn1 -- temp_Cell_B/RConn1 -- Temperature Sensor/LConn1
  Atmosphere Temperature/LConn1 -- Thermal Resistance/RConn1
  Jules Power Losses/RConn1 -- Simulink-PS Converter/RConn1
  PS-Simulink Converter/LConn1 -- Temperature Sensor/RConn2
  Thermal Reference/LConn1 -- Jules Power Losses/RConn2

== system Cooling_System/segment/Cell conductance2 ==
  Air-Iron Conductance : fl_lib/Thermal/Thermal Elements/Conductive Heat Transfer  area=0.014 m^2  thickness=2 mm  th_cond=0.0257 W/(m*K)  T_specify=off  T_priority=None  T=0 K  T_nominal_specify=off  T_nominal_unit=K  T_nominal_value=1  Q_specify=off  Q_priority=None  Q=0 W  Q_nominal_specify=off  Q_nominal_unit=W  Q_nominal_value=1
      settings: SourceProductName=Simscape
  Atmosphere Temperature : fl_lib/Thermal/Thermal Sources/Temperature Source  temperature=300 K
      settings: SourceProductName=Simscape
  Jules Power Losses : fl_lib/Thermal/Thermal Sources/Controlled Heat Flow Rate Source
      settings: SourceProductName=Simscape
  PS-Simulink Converter : nesl_utility/PS-Simulink Converter  PhysicalDomain=network_engine_domain  SubClassName=ps_output  LeftPortType=input  RightPortType=output  PseudoPeriodic=off  Frequencies=[]  Unit=1  AffineConversion=off
  Simulink-PS Converter : nesl_utility/Simulink-PS Converter  PhysicalDomain=network_engine_domain  SubClassName=ps_input  LeftPortType=input  RightPortType=output  PseudoPeriodic=off  Frequencies=[]  NoiseDistribution=none  NoiseParameters=[]  Unit=W  AffineConversion=off  FilteringAndDerivatives=zero  SimscapeFilterOrder=1  InputFilterTimeConstant=.001  UdotUserProvided=[]
  Stator Iron Thermal Mass : fl_lib/Thermal/Thermal Elements/Thermal Mass  mass=0.3 kg  sp_heat=460 J/kg/K  T_specify=off  T_priority=High  T=300 K  T_nominal_specify=off  T_nominal_unit=K  T_nominal_value=1  Q_specify=off  Q_priority=None  Q=0 W  Q_nominal_specify=off  Q_nominal_unit=W  Q_nominal_value=1
  Temperature Sensor : fl_lib/Thermal/Thermal Sensors/Temperature Sensor
  Thermal Reference : fl_lib/Thermal/Thermal Elements/Thermal Reference
  Thermal Resistance : fl_lib/Thermal/Thermal Elements/Thermal Resistance  resistance=1/(1.006*1.202*0.028*50.4/60*1000) K/W  T_specify=off  T_priority=None  T=0 K  T_nominal_specify=off  T_nominal_unit=K  T_nominal_value=1  Q_specify=off  Q_priority=None  Q=0 W  Q_nominal_specify=off  Q_nominal_unit=W  Q_nominal_value=1
      settings: SourceProductName=Simscape  SourceProductBaseCode=SS
  temp_Cell_A : PMIOPort  Side=Left
  temp_Cell_B : PMIOPort  Port=2  Side=Right
  tag scope: temp_cell_02=global
  wires:
  [Q_cell] -> Simulink-PS Converter/1
  PS-Simulink Converter/1 -> [temp_cell_02]
  connections:
  Jules Power Losses/LConn1 -- temp_Cell_A/RConn1 -- Temperature Sensor/RConn1 -- Stator Iron Thermal Mass/LConn1 -- Air-Iron Conductance/LConn1
  Air-Iron Conductance/RConn1 -- Thermal Resistance/LConn1 -- temp_Cell_B/RConn1 -- Temperature Sensor/LConn1
  Atmosphere Temperature/LConn1 -- Thermal Resistance/RConn1
  Jules Power Losses/RConn1 -- Simulink-PS Converter/RConn1
  PS-Simulink Converter/LConn1 -- Temperature Sensor/RConn2
  Thermal Reference/LConn1 -- Jules Power Losses/RConn2

== system Cooling_System/segment/Cell conductance20 ==
  Air-Iron Conductance : fl_lib/Thermal/Thermal Elements/Conductive Heat Transfer  area=0.014 m^2  thickness=2 mm  th_cond=0.0257 W/(m*K)  T_specify=off  T_priority=None  T=0 K  T_nominal_specify=off  T_nominal_unit=K  T_nominal_value=1  Q_specify=off  Q_priority=None  Q=0 W  Q_nominal_specify=off  Q_nominal_unit=W  Q_nominal_value=1
      settings: SourceProductName=Simscape
  Atmosphere Temperature : fl_lib/Thermal/Thermal Sources/Temperature Source  temperature=300 K
      settings: SourceProductName=Simscape
  Jules Power Losses : fl_lib/Thermal/Thermal Sources/Controlled Heat Flow Rate Source
      settings: SourceProductName=Simscape
  PS-Simulink Converter : nesl_utility/PS-Simulink Converter  PhysicalDomain=network_engine_domain  SubClassName=ps_output  LeftPortType=input  RightPortType=output  PseudoPeriodic=off  Frequencies=[]  Unit=1  AffineConversion=off
  Simulink-PS Converter : nesl_utility/Simulink-PS Converter  PhysicalDomain=network_engine_domain  SubClassName=ps_input  LeftPortType=input  RightPortType=output  PseudoPeriodic=off  Frequencies=[]  NoiseDistribution=none  NoiseParameters=[]  Unit=W  AffineConversion=off  FilteringAndDerivatives=zero  SimscapeFilterOrder=1  InputFilterTimeConstant=.001  UdotUserProvided=[]
  Stator Iron Thermal Mass : fl_lib/Thermal/Thermal Elements/Thermal Mass  mass=0.3 kg  sp_heat=460 J/kg/K  T_specify=off  T_priority=High  T=300 K  T_nominal_specify=off  T_nominal_unit=K  T_nominal_value=1  Q_specify=off  Q_priority=None  Q=0 W  Q_nominal_specify=off  Q_nominal_unit=W  Q_nominal_value=1
  Temperature Sensor : fl_lib/Thermal/Thermal Sensors/Temperature Sensor
  Thermal Reference : fl_lib/Thermal/Thermal Elements/Thermal Reference
  Thermal Resistance : fl_lib/Thermal/Thermal Elements/Thermal Resistance  resistance=1/(1.006*1.202*0.028*50.4/60*1000) K/W  T_specify=off  T_priority=None  T=0 K  T_nominal_specify=off  T_nominal_unit=K  T_nominal_value=1  Q_specify=off  Q_priority=None  Q=0 W  Q_nominal_specify=off  Q_nominal_unit=W  Q_nominal_value=1
      settings: SourceProductName=Simscape  SourceProductBaseCode=SS
  temp_Cell_A : PMIOPort  Side=Left
  temp_Cell_B : PMIOPort  Port=2  Side=Right
  tag scope: temp_cell_20=global
  wires:
  [Q_cell] -> Simulink-PS Converter/1
  PS-Simulink Converter/1 -> [temp_cell_20]
  connections:
  Jules Power Losses/LConn1 -- temp_Cell_A/RConn1 -- Temperature Sensor/RConn1 -- Stator Iron Thermal Mass/LConn1 -- Air-Iron Conductance/LConn1
  Air-Iron Conductance/RConn1 -- Thermal Resistance/LConn1 -- temp_Cell_B/RConn1 -- Temperature Sensor/LConn1
  Atmosphere Temperature/LConn1 -- Thermal Resistance/RConn1
  Jules Power Losses/RConn1 -- Simulink-PS Converter/RConn1
  PS-Simulink Converter/LConn1 -- Temperature Sensor/RConn2
  Thermal Reference/LConn1 -- Jules Power Losses/RConn2

== system Cooling_System/segment/Cell conductance21 ==
  Air-Iron Conductance : fl_lib/Thermal/Thermal Elements/Conductive Heat Transfer  area=0.014 m^2  thickness=2 mm  th_cond=0.0257 W/(m*K)  T_specify=off  T_priority=None  T=0 K  T_nominal_specify=off  T_nominal_unit=K  T_nominal_value=1  Q_specify=off  Q_priority=None  Q=0 W  Q_nominal_specify=off  Q_nominal_unit=W  Q_nominal_value=1
      settings: SourceProductName=Simscape
  Atmosphere Temperature : fl_lib/Thermal/Thermal Sources/Temperature Source  temperature=300 K
      settings: SourceProductName=Simscape
  Jules Power Losses : fl_lib/Thermal/Thermal Sources/Controlled Heat Flow Rate Source
      settings: SourceProductName=Simscape
  PS-Simulink Converter : nesl_utility/PS-Simulink Converter  PhysicalDomain=network_engine_domain  SubClassName=ps_output  LeftPortType=input  RightPortType=output  PseudoPeriodic=off  Frequencies=[]  Unit=1  AffineConversion=off
  Simulink-PS Converter : nesl_utility/Simulink-PS Converter  PhysicalDomain=network_engine_domain  SubClassName=ps_input  LeftPortType=input  RightPortType=output  PseudoPeriodic=off  Frequencies=[]  NoiseDistribution=none  NoiseParameters=[]  Unit=W  AffineConversion=off  FilteringAndDerivatives=zero  SimscapeFilterOrder=1  InputFilterTimeConstant=.001  UdotUserProvided=[]
  Stator Iron Thermal Mass : fl_lib/Thermal/Thermal Elements/Thermal Mass  mass=0.3 kg  sp_heat=460 J/kg/K  T_specify=off  T_priority=High  T=300 K  T_nominal_specify=off  T_nominal_unit=K  T_nominal_value=1  Q_specify=off  Q_priority=None  Q=0 W  Q_nominal_specify=off  Q_nominal_unit=W  Q_nominal_value=1
  Temperature Sensor : fl_lib/Thermal/Thermal Sensors/Temperature Sensor
  Thermal Reference : fl_lib/Thermal/Thermal Elements/Thermal Reference
  Thermal Resistance : fl_lib/Thermal/Thermal Elements/Thermal Resistance  resistance=1/(1.006*1.202*0.028*50.4/60*1000) K/W  T_specify=off  T_priority=None  T=0 K  T_nominal_specify=off  T_nominal_unit=K  T_nominal_value=1  Q_specify=off  Q_priority=None  Q=0 W  Q_nominal_specify=off  Q_nominal_unit=W  Q_nominal_value=1
      settings: SourceProductName=Simscape  SourceProductBaseCode=SS
  temp_Cell_A : PMIOPort  Side=Left
  temp_Cell_B : PMIOPort  Port=2  Side=Right
  tag scope: temp_cell_21=global
  wires:
  [Q_cell] -> Simulink-PS Converter/1
  PS-Simulink Converter/1 -> [temp_cell_21]
  connections:
  Jules Power Losses/LConn1 -- temp_Cell_A/RConn1 -- Temperature Sensor/RConn1 -- Stator Iron Thermal Mass/LConn1 -- Air-Iron Conductance/LConn1
  Air-Iron Conductance/RConn1 -- Thermal Resistance/LConn1 -- temp_Cell_B/RConn1 -- Temperature Sensor/LConn1
  Atmosphere Temperature/LConn1 -- Thermal Resistance/RConn1
  Jules Power Losses/RConn1 -- Simulink-PS Converter/RConn1
  PS-Simulink Converter/LConn1 -- Temperature Sensor/RConn2
  Thermal Reference/LConn1 -- Jules Power Losses/RConn2

== system Cooling_System/segment/Cell conductance22 ==
  Air-Iron Conductance : fl_lib/Thermal/Thermal Elements/Conductive Heat Transfer  area=0.014 m^2  thickness=2 mm  th_cond=0.0257 W/(m*K)  T_specify=off  T_priority=None  T=0 K  T_nominal_specify=off  T_nominal_unit=K  T_nominal_value=1  Q_specify=off  Q_priority=None  Q=0 W  Q_nominal_specify=off  Q_nominal_unit=W  Q_nominal_value=1
      settings: SourceProductName=Simscape
  Atmosphere Temperature : fl_lib/Thermal/Thermal Sources/Temperature Source  temperature=300 K
      settings: SourceProductName=Simscape
  Jules Power Losses : fl_lib/Thermal/Thermal Sources/Controlled Heat Flow Rate Source
      settings: SourceProductName=Simscape
  PS-Simulink Converter : nesl_utility/PS-Simulink Converter  PhysicalDomain=network_engine_domain  SubClassName=ps_output  LeftPortType=input  RightPortType=output  PseudoPeriodic=off  Frequencies=[]  Unit=1  AffineConversion=off
  Simulink-PS Converter : nesl_utility/Simulink-PS Converter  PhysicalDomain=network_engine_domain  SubClassName=ps_input  LeftPortType=input  RightPortType=output  PseudoPeriodic=off  Frequencies=[]  NoiseDistribution=none  NoiseParameters=[]  Unit=W  AffineConversion=off  FilteringAndDerivatives=zero  SimscapeFilterOrder=1  InputFilterTimeConstant=.001  UdotUserProvided=[]
  Stator Iron Thermal Mass : fl_lib/Thermal/Thermal Elements/Thermal Mass  mass=0.3 kg  sp_heat=460 J/kg/K  T_specify=off  T_priority=High  T=300 K  T_nominal_specify=off  T_nominal_unit=K  T_nominal_value=1  Q_specify=off  Q_priority=None  Q=0 W  Q_nominal_specify=off  Q_nominal_unit=W  Q_nominal_value=1
  Temperature Sensor : fl_lib/Thermal/Thermal Sensors/Temperature Sensor
  Thermal Reference : fl_lib/Thermal/Thermal Elements/Thermal Reference
  Thermal Resistance : fl_lib/Thermal/Thermal Elements/Thermal Resistance  resistance=1/(1.006*1.202*0.028*50.4/60*1000) K/W  T_specify=off  T_priority=None  T=0 K  T_nominal_specify=off  T_nominal_unit=K  T_nominal_value=1  Q_specify=off  Q_priority=None  Q=0 W  Q_nominal_specify=off  Q_nominal_unit=W  Q_nominal_value=1
      settings: SourceProductName=Simscape  SourceProductBaseCode=SS
  temp_Cell_A : PMIOPort  Side=Left
  temp_Cell_B : PMIOPort  Port=2  Side=Right
  tag scope: temp_cell_22=global
  wires:
  [Q_cell] -> Simulink-PS Converter/1
  PS-Simulink Converter/1 -> [temp_cell_22]
  connections:
  Jules Power Losses/LConn1 -- temp_Cell_A/RConn1 -- Temperature Sensor/RConn1 -- Stator Iron Thermal Mass/LConn1 -- Air-Iron Conductance/LConn1
  Air-Iron Conductance/RConn1 -- Thermal Resistance/LConn1 -- temp_Cell_B/RConn1 -- Temperature Sensor/LConn1
  Atmosphere Temperature/LConn1 -- Thermal Resistance/RConn1
  Jules Power Losses/RConn1 -- Simulink-PS Converter/RConn1
  PS-Simulink Converter/LConn1 -- Temperature Sensor/RConn2
  Thermal Reference/LConn1 -- Jules Power Losses/RConn2
